simulink model "NeuromorphicDogGait_WalksBackwards"  (R2022b)
settings: Solver=ode4  StartTime=0.0  StopTime=10  FixedStep=1e-3  RelTol=1e-3
undefined symbols (not defined in the file): t1, t2, Vus0
libraries: vexv5lib x24, vexcommonlib x16, Vex_V5_Simulink_Expansion x8
(part 3 of 3)

== matlab function NeuromorphicDogGait_WalksBackwards/Quad-Centre (Closed Coupling) Oscillator/QuadCentre (Closed) CPG/HalfCentre CPG P/MQIF_Neuron B/MATLAB Function1 ==
  data: State input; Derivatives output; I_ext input; excitatory_Vin input; inhibitory_Vin input; Params input
% This fcn implements the MQIF dynamics as ordinary differential equations.

function Derivatives = ODE(State, I_ext, excitatory_Vin, inhibitory_Vin, Params)
    % Parse through states
    V = State(1);
    Vs = State(2);
    Vus = State(3);
    Se = State(4:numel(excitatory_Vin)+3);
    Si = State(numel(excitatory_Vin)+4:end);

    % Parse through parameters
    g_f = Params(1);
    g_s = Params(2);
    g_us = Params(3);
    C = Params(4);
    tau_s = Params(5);
    tau_us = Params(6);
    tau_syn_E = Params(7);
    tau_syn_I = Params(8);
    Ve_syn = Params(9);
    Vi_syn = Params(10);
    g_syn_E = Params(11);
    g_syn_I = Params(12);
    Vin_gate_E = Params(13);
    Vin_gate_I = Params(14);
    k = Params(15);
    R = Params(16);
    V0 = Params(17);
    Vs0 = Params(18);
    Vus0 = Params(19);

    % Non-linear function to control synaptic gating
    sigmoid_Ve = 1./(1+exp(-(40*(excitatory_Vin-Vin_gate_E))));
    sigmoid_Vi = 1./(1+exp(-(40*(inhibitory_Vin-Vin_gate_I))));

    % Excitatory and inhibitory currents
    I_excitatory = g_syn_E*Se*(Ve_syn-V);
    I_inhibitory = g_syn_I*Si*(Vi_syn-V);

    % Passive Conductance in QuadCentre!!
    I_pass = (1/R)*(V-inhibitory_Vin(end-1));

    % ODE's that will be solved by the integrator block following this fcn
    V_dot = k*(((I_ext + g_f*((V-V0)^2) - g_s*((Vs-Vs0)^2) - g_us*((Vus-Vus0)^2) + sum(I_excitatory) + sum(I_inhibitory) + I_pass) / C));
    Vs_dot = k*((V - Vs) / tau_s);
    Vus_dot = k*((V - Vus) / tau_us);
    Se_dot = k*((sigmoid_Ve - Se)/tau_syn_E);
    Si_dot = k*((sigmoid_Vi - Si)/tau_syn_I);

    Derivatives = [V_dot; Vs_dot; Vus_dot; Se_dot; Si_dot];
end

== matlab function NeuromorphicDogGait_WalksBackwards/Quad-Centre (Closed Coupling) Oscillator/MQIF_Neuron Range of Motion Bounder A/MATLAB Function ==
  data: States input; reset output; V_threshold input
function reset = ResetTrigger(States, V_threshold)

V = States(1);

reset = (V > V_threshold);

end

== matlab function NeuromorphicDogGait_WalksBackwards/Quad-Centre (Closed Coupling) Oscillator/MQIF_Neuron Range of Motion Bounder A/MATLAB Function1 ==
  data: State input; Derivatives output; I_ext input; excitatory_Vin input; inhibitory_Vin input; Params input
function Derivatives = ODE(State, I_ext, excitatory_Vin, inhibitory_Vin, Params)
    V = State(1);
    Vs = State(2);
    Vus = State(3);
    Se = State(4);
    Si = State(5);

    g_f = Params(1);
    g_s = Params(2);
    g_us = Params(3);
    C = Params(4);
    tau_s = Params(5);
    tau_us = Params(6);
    tau_syn_E = Params(7);
    tau_syn_I = Params(8);
    Ve_syn = Params(9);
    Vi_syn = Params(10);
    g_syn_E = Params(11);
    g_syn_I = Params(12);
    Vin_gate_E = Params(13);
    Vin_gate_I = Params(14);
    k = Params(15);
    V0 = Params(16);
    Vs0 = Params(17);
    Vus0 = Params(18);
  
    sigmoid_Ve = 1/(1+exp(-(40*(sum(excitatory_Vin)-Vin_gate_E))));
    sigmoid_Vi = 1/(1+exp(-(40*(sum(inhibitory_Vin)-Vin_gate_I))));
    
    V_dot = k*(((I_ext + g_f*((V-V0)^2) - g_s*((Vs-Vs0)^2) - g_us*((Vus-Vus0)^2) + g_syn_E*Se*(Ve_syn-V) +g_syn_I*Si*(Vi_syn-V)) / C));
    Vs_dot = k*((V - Vs) / tau_s);
    Vus_dot = k*((V - Vus) / tau_us);
    Se_dot = k*((sigmoid_Ve - Se)/tau_syn_E);
    Si_dot = k*((sigmoid_Vi - Si)/tau_syn_I);

    Derivatives = [V_dot; Vs_dot; Vus_dot; Se_dot; Si_dot];
end

== matlab function NeuromorphicDogGait_WalksBackwards/Quad-Centre (Closed Coupling) Oscillator/QuadCentre (Closed) CPG/HalfCentre CPG P/MQIF_Neuron B/MATLAB Function2 ==
  data: inputVector input; outputVector output
% This function is required to make sure that the MQIF neuron is input
% agnostic, (can handle any number of excitatory/inhibitory connections).
% 
% We require a matrix that can extract Vus (scalar), Se and Si (vectors of
% arbitrary length), and ignore the other values. This is because these
% values are "remembered" after each action potential and are required in
% the subsequent resetting of states.

function outputVector = generalisedMatrix(inputVector)
    % Get the size of the input vector
    n = length(inputVector);

    % Create a square matrix of zeros
    Matrix = zeros(n);

    % Set the (3, 3) element to 1
    Matrix(3, 3) = 1;

    % Set the values for every row i, starting from the fourth row
    for i = 4:n
        Matrix(i, i) = 1;
    end

    outputVector = Matrix*inputVector;
end

== matlab function NeuromorphicDogGait_WalksBackwards/Quad-Centre (Closed Coupling) Oscillator/Lower Pain Function 2 ==
  data: params input; x input; y output
function y =  LowerRangeofMotion(params, x)
    c = params(1);
    u=params(2);
    
    y = 50/(1+exp(-u*(-x-c)));
end
